simulink model "lab3CTSys1"  (Simulink 4.00)
settings: Solver=ode45  SolverMode=SingleTasking  StartTime=0.0  StopTime=9999.0  MaxStep=.01  RelTol=1e-6  AbsTol=1e-6
settings Model: Creator=vise  LastModifiedBy=vise  InitialStep=.0001  LimitDataPoints=off  RTWTemplateMakefile=grt_unix.tmf  ExtModeTrigMode=oneshot  ExtModeArmWhenConnect=off  ExtModeAutoUpdateStatusClock=off

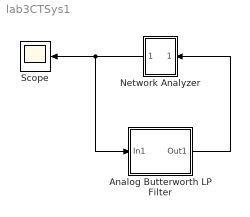
== system lab3CTSys1 ==
  Analog Butterworth LP Filter : Subsystem  mask(buttap){@1=2*pi, @2=4}
      mask prompts: @1 "Cutoff frequency (rad/sec)"; @2 "Order"
      mask help:
      | Analog Butterworth low pass filter.
      |
      | (Requires Signal Processing Toolbox)
      mask init:
      | [z,p,k]=buttap(@2); z=@1*z; p=@1*p; k=real(prod(-p)); [num,den]=zp2tf(z,p,k); w=logspace(log10(@1/10),log10(10*@1),20); h=freqs(num,den,w);
      settings: RTWFcnNameOpts=Auto  RTWFileNameOpts=Auto
      mask Help: Butterworth low pass filter using MATLAB's butter command.
      mask Display: plot(20*log10(w),20*log10(abs(h)))
  Network Analyzer : Subsystem  Orientation=left  mask(Network Analyzer){@1=256, @2=0.1}
      mask prompts: @1 "Number of sample points:"; @2 "Sampling period (sec):"
      mask init:
      | max_freq=0.9*pi/@2;N=@1;T_s=@2;const=2*pi/(@1*@2);window1=0.5*@1*@2;window2=@1*@2;
      settings: RTWFcnNameOpts=Auto  RTWFileNameOpts=Auto
      mask Help: Estimates frequency response of system using chirp input. Used for EE438. See Prof. Bouman.
      mask Display: plot(0,0,100,100,[11,93,93,11,11],[90,90,40,40,90],[80,60,40,20],[50,79,50,80])
  Scope : Scope
      settings: TickLabels=on  TimeRange=30  YMin=-1  YMax=1  SaveToWorkspace=off  SaveName=ScopeData  DataFormat=Array  LimitDataPoints=on  MaxDataPoints=5000
  wires:
  Network Analyzer/1(Outport) -> Scope/1, Analog Butterworth LP Filter/1(In1)
  Analog Butterworth LP Filter/1(Out1) -> Network Analyzer/1(Inport)

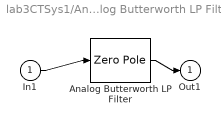
== system lab3CTSys1/Analog Butterworth LP Filter ==
  In1 : Inport  Port=1  LatchInput=off
  Analog Butterworth LP Filter : ZeroPole  Zeros=z  Poles=p  Gain=k  AbsoluteTolerance=auto
  Out1 : Outport  Port=1
  wires:
  In1/1 -> Analog Butterworth LP Filter/1
  Analog Butterworth LP Filter/1 -> Out1/1

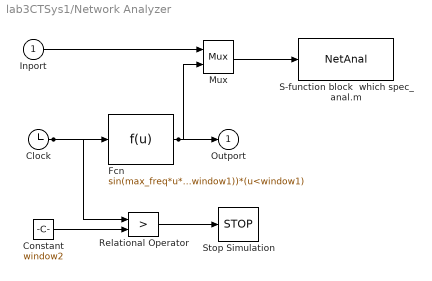
== system lab3CTSys1/Network Analyzer ==
  Inport : Inport  Port=1  LatchInput=off
  Clock : Clock
      settings: DisplayTime=off  Decimation=10
  Constant : Constant  Value=window2
  Fcn : Fcn  Expr=sin(max_freq*u*u/(2*window1))*(0.54+0.46*cos(pi*u/window1))*(u<window1)
  Mux : Mux  Inputs=2
      settings: DisplayOption=none
  Relational Operator : RelationalOperator  Operator=>
  S-function block  which spec_anal.m : S-Function  FunctionName=NetAnal  Parameters=N,T_s  PortCounts=[]  SFunctionModules=''
  Stop Simulation : Stop
  Outport : Outport  Port=1  InitialOutput=0
  wires:
  Relational Operator/1 -> Stop Simulation/1
  Constant/1 -> Relational Operator/2
  Clock/1 -> Relational Operator/1, Fcn/1
  Mux/1 -> S-function block  which spec_anal.m/1
  Fcn/1 -> Outport/1, Mux/2
  Inport/1 -> Mux/1
